simulink model "inv_pendel2"  (Simulink 4.00)
settings: Solver=ode45  StartTime=0.0  StopTime=10.0  RelTol=1e-3
values from neighbouring files (symbols this model uses):
  a = [-0.0558 -0.9968  0.0802 0.0415 ... (first row only)    [dynamik2.m]    (also in inv_pendel_1.m = [0,1,0,0;(M+m)*g/(M*l),0,0,0;0,0,0,1;-m*g/M,0,0,0]; inv_pendel_2.m = [0,1,0,0;(M+m)*g/(M*l),0,0,0;0,0,0,1;-m*g/M,0,0,0]; inv_pendel_3.m = [0,1,0,0;(M+m)*g/(M*l),0,0,0;0,0,0,1;-m*g/M,0,0,0]; inv_pendel_4.m = [0,1,0,0;(M+m)*g/(M*l),0,0,0;0,0,0,1;-m*g/M,0,0,0])
  b = [0.0073 0 ... (first row only)    [dynamik2.m]    (also in inv_pendel_1.m = [0,-1/(M*l),0,1/M]'; inv_pendel_2.m = [0,-1/(M*l),0,1/M]'; inv_pendel_3.m = [0,-1/(M*l),0,1/M]'; inv_pendel_4.m = [0,-1/(M*l),0,1/M]')
  c = 8.8e5    (= 880000)    [bohrhammer1.m]    (also in bohrhammer2.m; dynamik2.m = [0 1 0 0; inv_pendel_1.m = [1,0,0,0;0,0,1,0]; inv_pendel_2.m = eye(4,4))
  d = 22.2    [bohrhammer1.m]    (also in bohrhammer2.m; dynamik2.m = [0 0;0 0]; inv_pendel_1.m = 0; inv_pendel_2.m = zeros(4,1))
  K = place(a,b,p)    [inv_pendel_2.m]    (also in inv_pendel_3.m; inv_pendel_4.m; zeitdiskret_1.m = [1,0;10,1])
settings Model: LastModifiedBy=Administrator  BlockReductionOpt=off

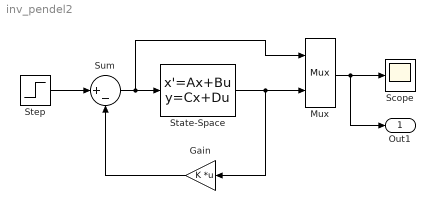
== system inv_pendel2 ==
  Gain : Gain  Orientation=left  Gain=K  Multiplication=Matrix(K*u)  SaturateOnIntegerOverflow=on
  Mux : Mux  Inputs=2
      settings: DisplayOption=none
  Scope : Scope
      settings: TimeRange=auto  YMin=-5  YMax=5  SaveToWorkspace=off  SaveName=ScopeData  LimitDataPoints=on  MaxDataPoints=5000
  State-Space : StateSpace  A=a  B=b  C=c  D=d  X0=0  Realization=auto  AbsoluteTolerance=auto
  Step : Step  Time=0  Before=0  After=1  SampleTime=0
  Sum : Sum  Inputs=|+-  SaturateOnIntegerOverflow=on
  Out1 : Outport  Port=1
  wires:
  Sum/1 -> State-Space/1, Mux/1
  Step/1 -> Sum/1
  State-Space/1 -> Gain/1, Mux/2
  Gain/1 -> Sum/2
  Mux/1 -> Scope/1, Out1/1
